simulink library "Aerodynamics"  (R2024b)
settings: Solver=VariableStepAuto  StartTime=0.0  StopTime=10.0  RelTol=1e-3
undefined symbols (not defined in the file): b, c, CD0, CD_alpha, CD_elev, CL0, Cl_ail, CL_alpha, CL_AlphaDot, Cl_beta, CL_elev, Cl_p, CL_q, Cl_r, Cl_rud, Cm0, Cm_alpha, Cm_AlphaDot, Cm_elev, Cm_q, Cn_ail, Cn_beta, Cn_p, Cn_r, Cn_rud, CY_ail, CY_beta, CY_p, CY_r, CY_rud, S, y_cg, z_cg
settings Model: Creator=ada09  LastModifiedBy=ada09

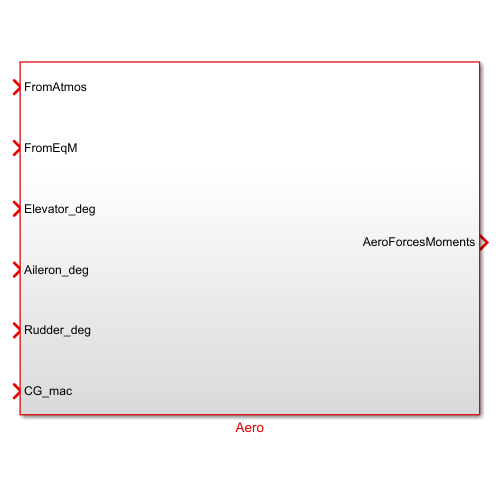
[thumbnail: Simulink's stored preview of the top-level diagram]
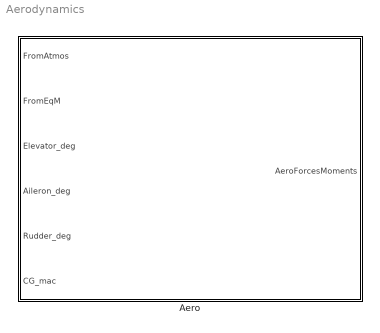
== system Aerodynamics ==
  Aero : Subsystem

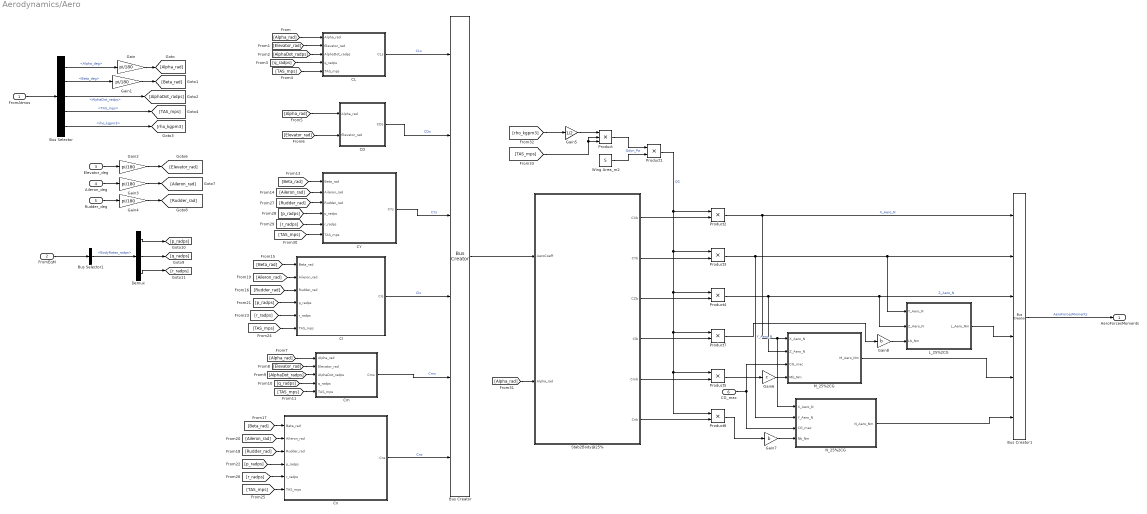
== system Aerodynamics/Aero ==
  FromAtmos : Inport
  FromEqM : Inport  Port=2
  Elevator_deg : Inport  Port=3
  Aileron_deg : Inport  Port=4
  Rudder_deg : Inport  Port=5
  CG_mac : Inport  Port=6
  Bus Creator : BusCreator  Inputs=6
  Bus Creator1 : BusCreator  Inputs=6
  Bus Selector : BusSelector  OutputSignals=Alpha_deg,Beta_deg,AlphaDot_radps,TAS_mps,rho_kgpm3
  Bus Selector1 : BusSelector  OutputSignals=BodyRates_radps
  CD : Subsystem
  CL : Subsystem
  CY : Subsystem
  Cl : Subsystem
  Cm : Subsystem
  Cn : Subsystem
  Demux : Demux  Outputs=3
  Gain{,1..4} (5 alike) : Gain  Gain=pi/180
  Gain5 : Gain  Gain=1/2
  Gain6 : Gain  Gain=c
  Gain7 : Gain  Gain=b
  Gain8 : Gain  Gain=b
  L_25%2CG : Subsystem
  M_25%2CG : Subsystem
  N_25%2CG : Subsystem
  Product : Product  Inputs=3
  Product{1..7} (7 alike) : Product
  Stab2Body@25% : Subsystem
  Wing Area_m2 : Constant  Value=S
  AeroForcesMoments : Outport
  wires:
  Bus Selector1/1 -> Demux/1  "<BodyRates_radps>"
  Bus Selector/1 -> Gain/1  "<Alpha_deg>"
  Bus Selector/3 -> [AlphaDot_radps]  "<AlphaDot_radps>"
  Bus Selector/2 -> Gain1/1  "<Beta_deg>"
  Bus Selector/4 -> [TAS_mps]  "<TAS_mps>"
  Bus Selector/5 -> [rho_kgpm3]  "<rho_kgpm3>"
  FromEqM/1 -> Bus Selector1/1
  FromAtmos/1 -> Bus Selector/1
  Stab2Body@25%/4(Clb) -> Product7/2
  Stab2Body@25%/1(CXb) -> Product2/2
  [Aileron_rad] -> Cl/2(Aileron_rad)
  Demux/3 -> [r_radps]
  [Elevator_rad] -> CL/2(Elevator_rad)
  Product/1 -> Product1/1  "Qdyn_Pa"
  [AlphaDot_radps] -> CL/3(AlphaDot_radps)
  [Rudder_rad] -> CY/3(Rudder_rad)
  [TAS_mps] -> Product/2, Product/3
  Gain6/1 -> M_25%2CG/4(Mb_Nm)
  [rho_kgpm3] -> Gain5/1
  [Aileron_rad] -> CY/2(Aileron_rad)
  Bus Creator/1 -> Stab2Body@25%/1(AeroCoeff)
  [TAS_mps] -> CL/5(TAS_mps)
  Rudder_deg/1 -> Gain4/1
  Stab2Body@25%/2(CYb) -> Product3/2
  [Beta_rad] -> Cl/1(Beta_rad)
  [r_radps] -> Cn/5(r_radps)
  Demux/2 -> [q_radps]
  [p_radps] -> CY/4(p_radps)
  [Alpha_rad] -> Cm/1(Alpha_rad)
  Aileron_deg/1 -> Gain3/1
  Gain4/1 -> [Rudder_rad]
  Gain8/1 -> L_25%2CG/3(Lb_Nm)
  [Alpha_rad] -> CD/1(Alpha_rad)
  [AlphaDot_radps] -> Cm/3(AlphaDot_radps)
  Stab2Body@25%/3(CZb) -> Product4/2
  CL/1(CLs) -> Bus Creator/1  "CLs"
  Elevator_deg/1 -> Gain2/1
  [TAS_mps] -> Cm/5(TAS_mps)
  [r_radps] -> Cl/5(r_radps)
  Gain3/1 -> [Aileron_rad]
  Gain/1 -> [Alpha_rad]
  [p_radps] -> Cn/4(p_radps)
  Product2/1 -> M_25%2CG/1(X_Aero_N), N_25%2CG/1(X_Aero_N), Bus Creator1/1  "X_Aero_N"
  Product3/1 -> N_25%2CG/2(Y_Aero_N), L_25%2CG/1(Y_Aero_N), Bus Creator1/2  "Y_Aero_N"
  Stab2Body@25%/6(Cnb) -> Product6/2
  Gain1/1 -> [Beta_rad]
  [Elevator_rad] -> CD/2(Elevator_rad)
  Wing Area_m2/1 -> Product1/2
  Gain5/1 -> Product/1
  Product4/1 -> M_25%2CG/2(Z_Aero_N), Bus Creator1/3, L_25%2CG/2(Z_Aero_N)  "Z_Aero_N"
  Gain2/1 -> [Elevator_rad]
  [Alpha_rad] -> CL/1(Alpha_rad)
  [Elevator_rad] -> Cm/2(Elevator_rad)
  Product1/1 -> Product4/1, Product7/1, Product6/1, Product5/1, Product3/1, Product2/1  "QS"
  [p_radps] -> Cl/4(p_radps)
  CG_mac/1 -> N_25%2CG/3(CG_mac), M_25%2CG/3(CG_mac)
  [Aileron_rad] -> Cn/2(Aileron_rad)
  Demux/1 -> [p_radps]
  Product5/1 -> Gain6/1
  [Beta_rad] -> CY/1(Beta_rad)
  [q_radps] -> Cm/4(q_radps)
  [Beta_rad] -> Cn/1(Beta_rad)
  [TAS_mps] -> Cl/6(TAS_mps)
  [Rudder_rad] -> Cl/3(Rudder_rad)
  [Rudder_rad] -> Cn/3(Rudder_rad)
  [q_radps] -> CL/4(q_radps)
  Product7/1 -> Gain8/1
  M_25%2CG/1(M_Aero_Nm) -> Bus Creator1/5
  [Alpha_rad] -> Stab2Body@25%/2(Alpha_rad)
  Cn/1(Cns) -> Bus Creator/6  "Cns"
  Gain7/1 -> N_25%2CG/4(Nb_Nm)
  Product6/1 -> Gain7/1
  [TAS_mps] -> Cn/6(TAS_mps)
  Cl/1(Cls) -> Bus Creator/4  "Cls"
  CY/1(CYs) -> Bus Creator/3  "CYs"
  CD/1(CDs) -> Bus Creator/2  "CDs"
  [r_radps] -> CY/5(r_radps)
  Cm/1(Cms) -> Bus Creator/5  "Cms"
  [TAS_mps] -> CY/6(TAS_mps)
  N_25%2CG/1(N_Aero_Nm) -> Bus Creator1/6
  Stab2Body@25%/5(Cmb) -> Product5/2
  L_25%2CG/1(L_Aero_Nm) -> Bus Creator1/4
  Bus Creator1/1 -> AeroForcesMoments/1  "AeroForcesMoments"

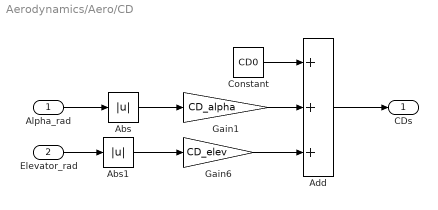
== system Aerodynamics/Aero/CD ==
  Alpha_rad : Inport
  Elevator_rad : Inport  Port=2
  Abs : Abs  SaturateOnIntegerOverflow=off
  Abs1 : Abs  SaturateOnIntegerOverflow=off
  Add : Sum  Inputs=+++
  Constant : Constant  Value=CD0
  Gain1 : Gain  Gain=CD_alpha
  Gain6 : Gain  Gain=CD_elev
  CDs : Outport
  wires:
  Constant/1 -> Add/1
  Gain6/1 -> Add/3
  Elevator_rad/1 -> Abs1/1
  Add/1 -> CDs/1
  Alpha_rad/1 -> Abs/1
  Abs/1 -> Gain1/1
  Gain1/1 -> Add/2
  Abs1/1 -> Gain6/1

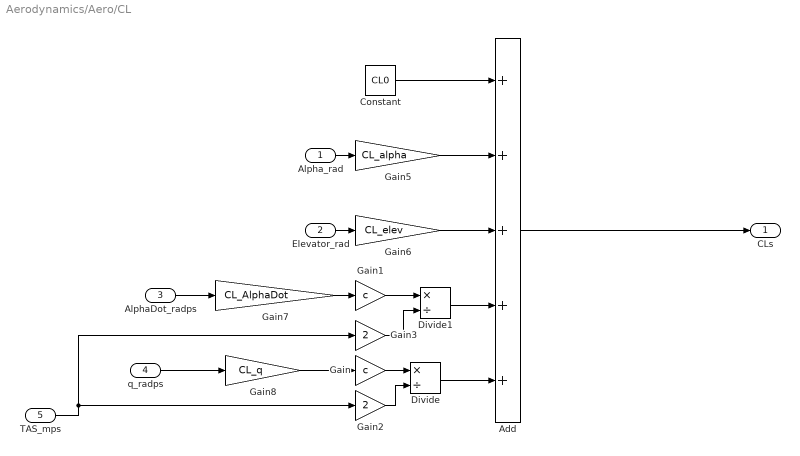
== system Aerodynamics/Aero/CL ==
  Alpha_rad : Inport
  Elevator_rad : Inport  Port=2
  AlphaDot_radps : Inport  Port=3
  q_radps : Inport  Port=4
  TAS_mps : Inport  Port=5
  Add : Sum  Inputs=+++++
  Constant : Constant  Value=CL0
  Divide : Product  Inputs=*/
  Divide1 : Product  Inputs=*/
  Gain : Gain  Gain=c
  Gain1 : Gain  Gain=c
  Gain2 : Gain  Gain=2
  Gain3 : Gain  Gain=2
  Gain5 : Gain  Gain=CL_alpha
  Gain6 : Gain  Gain=CL_elev
  Gain7 : Gain  Gain=CL_AlphaDot
  Gain8 : Gain  Gain=CL_q
  CLs : Outport
  wires:
  Constant/1 -> Add/1
  q_radps/1 -> Gain8/1
  Gain8/1 -> Gain/1
  Alpha_rad/1 -> Gain5/1
  Gain6/1 -> Add/3
  Gain5/1 -> Add/2
  Gain7/1 -> Gain1/1
  Elevator_rad/1 -> Gain6/1
  AlphaDot_radps/1 -> Gain7/1
  Add/1 -> CLs/1
  Gain/1 -> Divide/1
  Divide/1 -> Add/5
  TAS_mps/1 -> Gain3/1, Gain2/1
  Gain2/1 -> Divide/2
  Gain1/1 -> Divide1/1
  Divide1/1 -> Add/4
  Gain3/1 -> Divide1/2

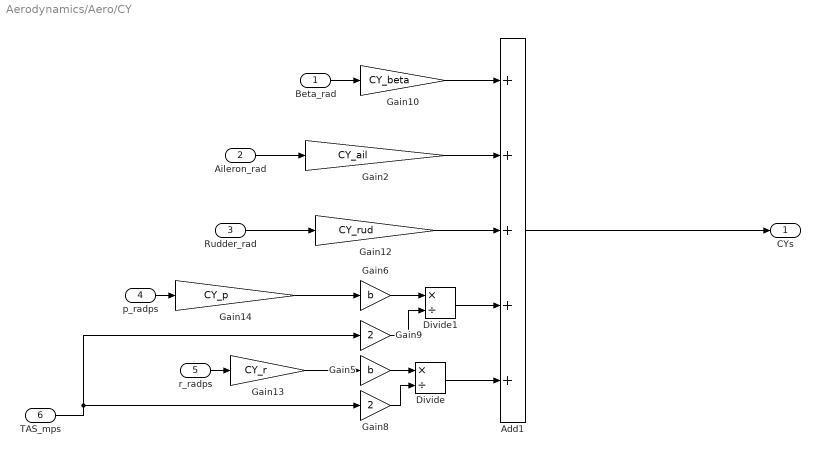
== system Aerodynamics/Aero/CY ==
  Beta_rad : Inport
  Aileron_rad : Inport  Port=2
  Rudder_rad : Inport  Port=3
  p_radps : Inport  Port=4
  r_radps : Inport  Port=5
  TAS_mps : Inport  Port=6
  Add1 : Sum  Inputs=+++++
  Divide : Product  Inputs=*/
  Divide1 : Product  Inputs=*/
  Gain10 : Gain  Gain=CY_beta
  Gain12 : Gain  Gain=CY_rud
  Gain13 : Gain  Gain=CY_r
  Gain14 : Gain  Gain=CY_p
  Gain2 : Gain  Gain=CY_ail
  Gain5 : Gain  Gain=b
  Gain6 : Gain  Gain=b
  Gain8 : Gain  Gain=2
  Gain9 : Gain  Gain=2
  CYs : Outport
  wires:
  p_radps/1 -> Gain14/1
  Rudder_rad/1 -> Gain12/1
  Divide1/1 -> Add1/4
  r_radps/1 -> Gain13/1
  Gain5/1 -> Divide/1
  Gain9/1 -> Divide1/2
  Beta_rad/1 -> Gain10/1
  Add1/1 -> CYs/1
  Gain8/1 -> Divide/2
  Gain13/1 -> Gain5/1
  Divide/1 -> Add1/5
  TAS_mps/1 -> Gain9/1, Gain8/1
  Gain12/1 -> Add1/3
  Gain10/1 -> Add1/1
  Gain6/1 -> Divide1/1
  Gain14/1 -> Gain6/1
  Aileron_rad/1 -> Gain2/1
  Gain2/1 -> Add1/2

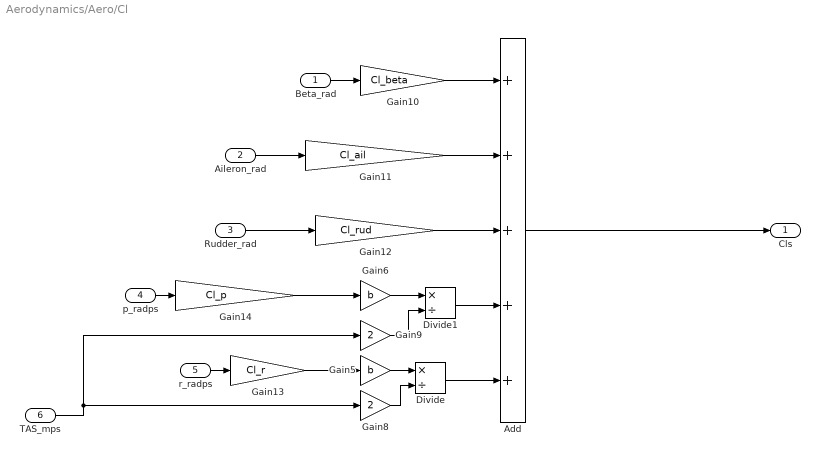
== system Aerodynamics/Aero/Cl ==
  Beta_rad : Inport
  Aileron_rad : Inport  Port=2
  Rudder_rad : Inport  Port=3
  p_radps : Inport  Port=4
  r_radps : Inport  Port=5
  TAS_mps : Inport  Port=6
  Add : Sum  Inputs=+++++
  Divide : Product  Inputs=*/
  Divide1 : Product  Inputs=*/
  Gain10 : Gain  Gain=Cl_beta
  Gain11 : Gain  Gain=Cl_ail
  Gain12 : Gain  Gain=Cl_rud
  Gain13 : Gain  Gain=Cl_r
  Gain14 : Gain  Gain=Cl_p
  Gain5 : Gain  Gain=b
  Gain6 : Gain  Gain=b
  Gain8 : Gain  Gain=2
  Gain9 : Gain  Gain=2
  Cls : Outport
  wires:
  Gain8/1 -> Divide/2
  Gain13/1 -> Gain5/1
  Gain6/1 -> Divide1/1
  Aileron_rad/1 -> Gain11/1
  Gain14/1 -> Gain6/1
  Gain12/1 -> Add/3
  TAS_mps/1 -> Gain9/1, Gain8/1
  Gain11/1 -> Add/2
  Gain10/1 -> Add/1
  Divide/1 -> Add/5
  Gain5/1 -> Divide/1
  Add/1 -> Cls/1
  Gain9/1 -> Divide1/2
  Beta_rad/1 -> Gain10/1
  Rudder_rad/1 -> Gain12/1
  Divide1/1 -> Add/4
  p_radps/1 -> Gain14/1
  r_radps/1 -> Gain13/1

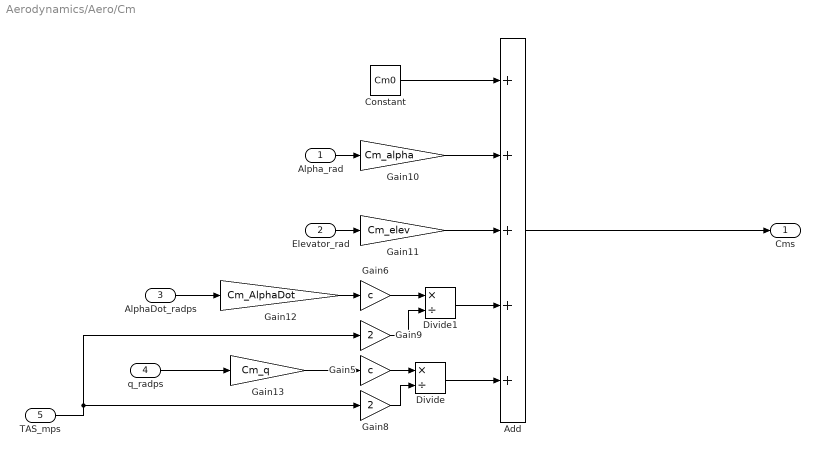
== system Aerodynamics/Aero/Cm ==
  Alpha_rad : Inport
  Elevator_rad : Inport  Port=2
  AlphaDot_radps : Inport  Port=3
  q_radps : Inport  Port=4
  TAS_mps : Inport  Port=5
  Add : Sum  Inputs=+++++
  Constant : Constant  Value=Cm0
  Divide : Product  Inputs=*/
  Divide1 : Product  Inputs=*/
  Gain10 : Gain  Gain=Cm_alpha
  Gain11 : Gain  Gain=Cm_elev
  Gain12 : Gain  Gain=Cm_AlphaDot
  Gain13 : Gain  Gain=Cm_q
  Gain5 : Gain  Gain=c
  Gain6 : Gain  Gain=c
  Gain8 : Gain  Gain=2
  Gain9 : Gain  Gain=2
  Cms : Outport
  wires:
  Gain13/1 -> Gain5/1
  Divide/1 -> Add/5
  TAS_mps/1 -> Gain9/1, Gain8/1
  Gain11/1 -> Add/3
  Gain8/1 -> Divide/2
  Alpha_rad/1 -> Gain10/1
  Gain9/1 -> Divide1/2
  Add/1 -> Cms/1
  Gain5/1 -> Divide/1
  q_radps/1 -> Gain13/1
  AlphaDot_radps/1 -> Gain12/1
  Gain12/1 -> Gain6/1
  Gain10/1 -> Add/2
  Constant/1 -> Add/1
  Gain6/1 -> Divide1/1
  Divide1/1 -> Add/4
  Elevator_rad/1 -> Gain11/1

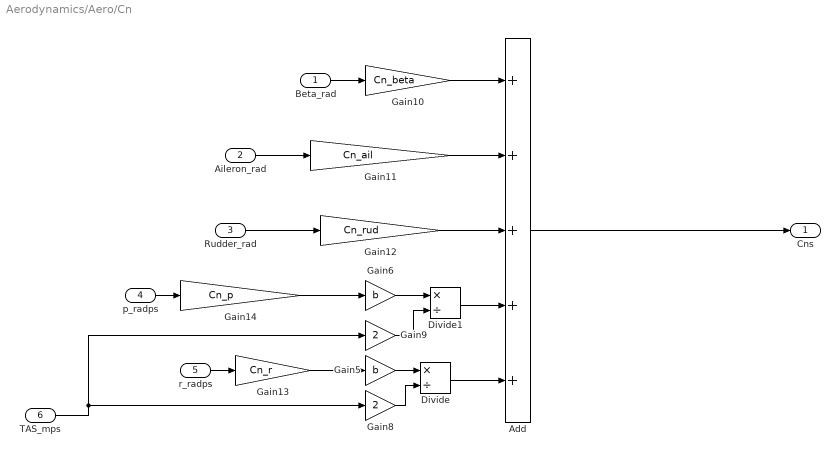
== system Aerodynamics/Aero/Cn ==
  Beta_rad : Inport
  Aileron_rad : Inport  Port=2
  Rudder_rad : Inport  Port=3
  p_radps : Inport  Port=4
  r_radps : Inport  Port=5
  TAS_mps : Inport  Port=6
  Add : Sum  Inputs=+++++
  Divide : Product  Inputs=*/
  Divide1 : Product  Inputs=*/
  Gain10 : Gain  Gain=Cn_beta
  Gain11 : Gain  Gain=Cn_ail
  Gain12 : Gain  Gain=Cn_rud
  Gain13 : Gain  Gain=Cn_r
  Gain14 : Gain  Gain=Cn_p
  Gain5 : Gain  Gain=b
  Gain6 : Gain  Gain=b
  Gain8 : Gain  Gain=2
  Gain9 : Gain  Gain=2
  Cns : Outport
  wires:
  Aileron_rad/1 -> Gain11/1
  Divide1/1 -> Add/4
  Gain10/1 -> Add/1
  Gain9/1 -> Divide1/2
  Beta_rad/1 -> Gain10/1
  TAS_mps/1 -> Gain9/1, Gain8/1
  Add/1 -> Cns/1
  Gain5/1 -> Divide/1
  r_radps/1 -> Gain13/1
  p_radps/1 -> Gain14/1
  Gain8/1 -> Divide/2
  Divide/1 -> Add/5
  Gain13/1 -> Gain5/1
  Rudder_rad/1 -> Gain12/1
  Gain6/1 -> Divide1/1
  Gain14/1 -> Gain6/1
  Gain12/1 -> Add/3
  Gain11/1 -> Add/2

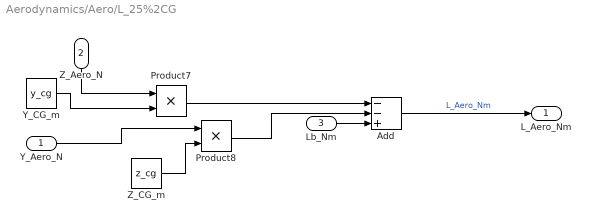
== system Aerodynamics/Aero/L_25%2CG ==
  Y_Aero_N : Inport
  Z_Aero_N : Inport  Port=2
  Lb_Nm : Inport  Port=3
  Add : Sum  Inputs=--+
  Product7 : Product
  Product8 : Product
  Y_CG_m : Constant  Value=y_cg
  Z_CG_m : Constant  Value=z_cg
  L_Aero_Nm : Outport
  wires:
  Product7/1 -> Add/1
  Y_Aero_N/1 -> Product8/1
  Z_Aero_N/1 -> Product7/1
  Lb_Nm/1 -> Add/3
  Add/1 -> L_Aero_Nm/1  "L_Aero_Nm"
  Product8/1 -> Add/2
  Z_CG_m/1 -> Product8/2
  Y_CG_m/1 -> Product7/2

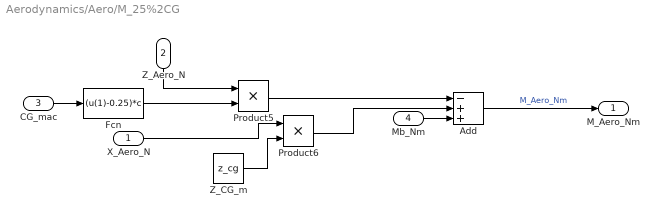
== system Aerodynamics/Aero/M_25%2CG ==
  X_Aero_N : Inport
  Z_Aero_N : Inport  Port=2
  CG_mac : Inport  Port=3
  Mb_Nm : Inport  Port=4
  Add : Sum  Inputs=-++
  Fcn : Fcn  Expr=(u(1)-0.25)*c
  Product5 : Product
  Product6 : Product
  Z_CG_m : Constant  Value=z_cg
  M_Aero_Nm : Outport
  wires:
  Product6/1 -> Add/2
  Mb_Nm/1 -> Add/3
  Add/1 -> M_Aero_Nm/1  "M_Aero_Nm"
  Fcn/1 -> Product5/2
  CG_mac/1 -> Fcn/1
  X_Aero_N/1 -> Product6/1
  Z_CG_m/1 -> Product6/2
  Product5/1 -> Add/1
  Z_Aero_N/1 -> Product5/1

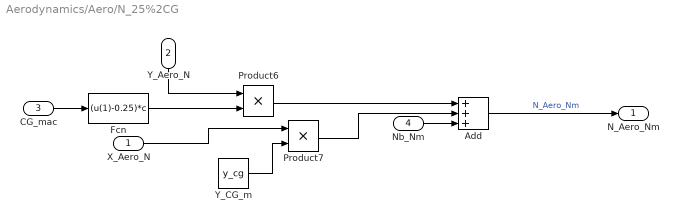
== system Aerodynamics/Aero/N_25%2CG ==
  X_Aero_N : Inport
  Y_Aero_N : Inport  Port=2
  CG_mac : Inport  Port=3
  Nb_Nm : Inport  Port=4
  Add : Sum  Inputs=+++
  Fcn : Fcn  Expr=(u(1)-0.25)*c
  Product6 : Product
  Product7 : Product
  Y_CG_m : Constant  Value=y_cg
  N_Aero_Nm : Outport
  wires:
  Nb_Nm/1 -> Add/3
  CG_mac/1 -> Fcn/1
  X_Aero_N/1 -> Product7/1
  Y_Aero_N/1 -> Product6/1
  Y_CG_m/1 -> Product7/2
  Product6/1 -> Add/1
  Add/1 -> N_Aero_Nm/1  "N_Aero_Nm"
  Fcn/1 -> Product6/2
  Product7/1 -> Add/2

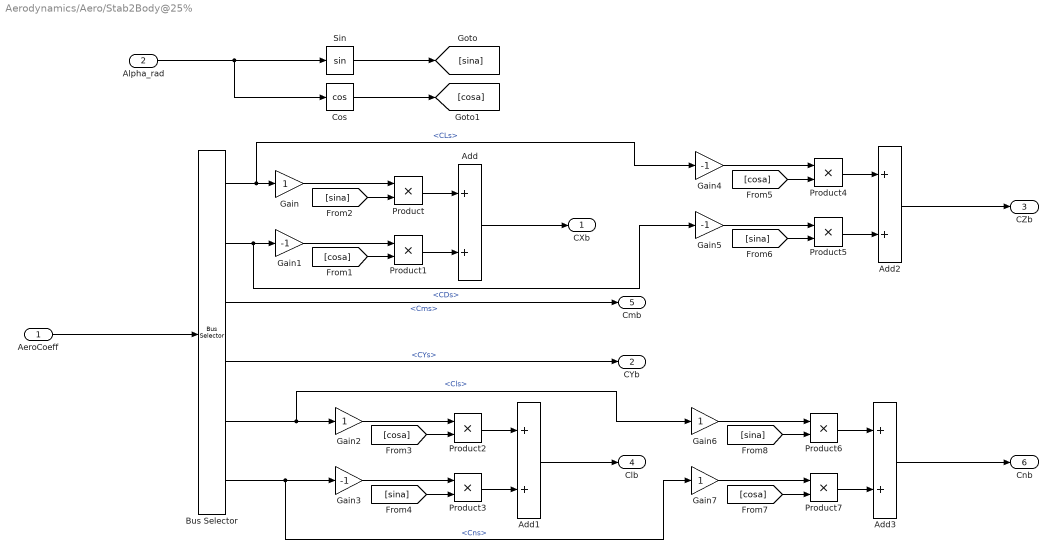
== system Aerodynamics/Aero/Stab2Body@25% ==
  AeroCoeff : Inport
  Alpha_rad : Inport  Port=2
  Add{,1..3} (4 alike) : Sum
  Bus Selector : BusSelector  OutputSignals=CLs,CDs,Cms,CYs,Cls,Cns
  Cos : Trigonometry  Operator=cos
  Gain{,2,6..7} (4 alike) : Gain
  Gain{1,3..5} (4 alike) : Gain  Gain=-1
  Product{,1..7} (8 alike) : Product
  Sin : Trigonometry
  CXb : Outport
  CYb : Outport  Port=2
  CZb : Outport  Port=3
  Clb : Outport  Port=4
  Cmb : Outport  Port=5
  Cnb : Outport  Port=6
  wires:
  AeroCoeff/1 -> Bus Selector/1
  Alpha_rad/1 -> Cos/1, Sin/1
  Sin/1 -> [sina]
  Cos/1 -> [cosa]
  Bus Selector/1 -> Gain4/1, Gain/1  "<CLs>"
  [sina] -> Product/2
  Bus Selector/2 -> Gain5/1, Gain1/1  "<CDs>"
  [cosa] -> Product1/2
  Product1/1 -> Add/2
  Product/1 -> Add/1
  Add/1 -> CXb/1
  Gain/1 -> Product/1
  Gain1/1 -> Product1/1
  Gain2/1 -> Product2/1
  Product3/1 -> Add1/2
  Product2/1 -> Add1/1
  Gain3/1 -> Product3/1
  Add1/1 -> Clb/1
  Bus Selector/3 -> Cmb/1  "<Cms>"
  Bus Selector/4 -> CYb/1  "<CYs>"
  Bus Selector/5 -> Gain6/1, Gain2/1  "<Cls>"
  [cosa] -> Product2/2
  [sina] -> Product3/2
  Gain4/1 -> Product4/1
  Product5/1 -> Add2/2
  Product4/1 -> Add2/1
  Gain5/1 -> Product5/1
  Add2/1 -> CZb/1
  [cosa] -> Product4/2
  [sina] -> Product5/2
  Bus Selector/6 -> Gain7/1, Gain3/1  "<Cns>"
  Product6/1 -> Add3/1
  Gain6/1 -> Product6/1
  Gain7/1 -> Product7/1
  Add3/1 -> Cnb/1
  Product7/1 -> Add3/2
  [sina] -> Product6/2
  [cosa] -> Product7/2
